simulink model "Subsystem"  (R2020b)
settings: Solver=FixedStepAuto  StartTime=0.0  StopTime=10.0  FixedStep=0.2  RelTol=1e-3
settings Model: Creator=ADMIN  LastModifiedBy=ADMIN
settings DataIOCC: SaveOutput=off  SaveTime=off

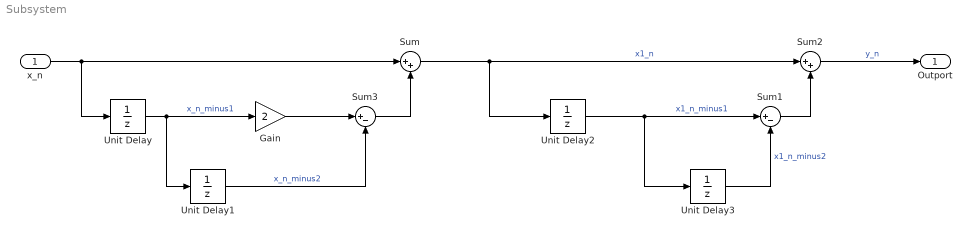
== system Subsystem ==
  x_n : Inport  OutDataTypeStr=double  PortDimensions=1  SampleTime=[0.20000000000000001,0]
  Gain : Gain  Gain=2
  Sum : Sum  Inputs=|++
  Sum1 : Sum  Inputs=|+-
  Sum2 : Sum  Inputs=|++
  Sum3 : Sum  Inputs=|+-
  Unit Delay{,1..3} (4 alike) : UnitDelay  SampleTime=-1  HasFrameUpgradeWarning=on
  Outport : Outport  OutDataTypeStr=double  PortDimensions=1  SampleTime=[0.20000000000000001,0]
  wires:
  Sum/1 -> Sum2/1, Unit Delay2/1  "x1_n"
  x_n/1 -> Sum/1, Unit Delay/1
  Sum1/1 -> Sum2/2
  Gain/1 -> Sum3/1
  Unit Delay2/1 -> Sum1/1, Unit Delay3/1  "x1_n_minus1"
  Unit Delay1/1 -> Sum3/2  "x_n_minus2"
  Unit Delay/1 -> Gain/1, Unit Delay1/1  "x_n_minus1"
  Sum2/1 -> Outport/1  "y_n"
  Unit Delay3/1 -> Sum1/2  "x1_n_minus2"
  Sum3/1 -> Sum/2
